simulink model "Zad1"  (R2020b)
settings: Solver=VariableStepAuto  StartTime=0.0  StopTime=0.0  RelTol=1e-3
libraries: CPOiS_SourcesSinks x10, CPOiS_DataManipulation x6, CPOiS_DataManipulation_DataTypeConversion x4, CPOiS_LinearTransforms x2, CPOiS_Filters x2, CPOiS_DataManipulation_IntroduceNoise x1, CPOiS_General x1
settings Model: Creator=Krystian  LastModifiedBy=Krystian

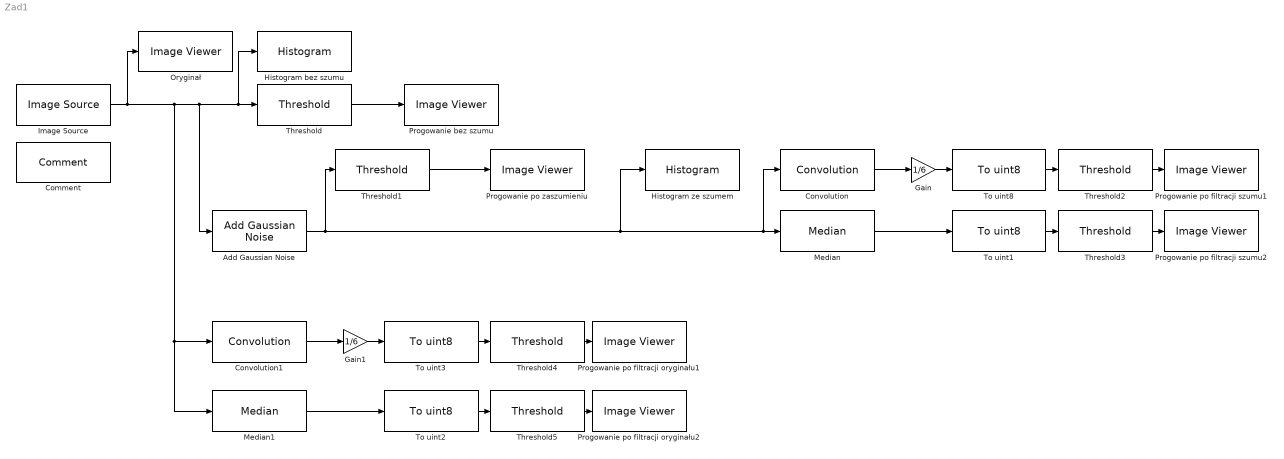
== system Zad1 ==
  Add Gaussian Noise : CPOiS_DataManipulation_IntroduceNoise/Add Gaussian Noise  Mean=0  Variance=1
      settings: SourceProductName=CPOiS - Digital image and signal processing
  Comment : CPOiS_General/Comment
      settings: SourceProductName=CPOiS - Digital image and signal processing
  Convolution : CPOiS_LinearTransforms/Convolution  ConvolutionMatrix=[0,1,0;1,2,1;0,1,0]
      settings: SourceProductName=CPOiS - Digital image and signal processing
  Convolution1 : CPOiS_LinearTransforms/Convolution  ConvolutionMatrix=[0,1,0;1,2,1;0,1,0]
      settings: SourceProductName=CPOiS - Digital image and signal processing
  Gain : Gain  Gain=1/6
  Gain1 : Gain  Gain=1/6
  Histogram bez szumu : CPOiS_SourcesSinks/Histogram
      settings: SourceProductName=CPOiS - Digital image and signal processing
  Histogram ze szumem : CPOiS_SourcesSinks/Histogram
      settings: SourceProductName=CPOiS - Digital image and signal processing
  Image Source : CPOiS_SourcesSinks/Image Source  FileSelection=cameraman.tif
      settings: SourceProductName=CPOiS - Digital image and signal processing
  Median : CPOiS_Filters/Median  MaskSize=3 x 3
      settings: SourceProductName=CPOiS - Digital image and signal processing
  Median1 : CPOiS_Filters/Median  MaskSize=3 x 3
      settings: SourceProductName=CPOiS - Digital image and signal processing
  Oryginał : CPOiS_SourcesSinks/Image Viewer
      settings: SourceProductName=CPOiS - Digital image and signal processing
  Progowanie bez szumu : CPOiS_SourcesSinks/Image Viewer
      settings: SourceProductName=CPOiS - Digital image and signal processing
  Progowanie po filtracji oryginału1 : CPOiS_SourcesSinks/Image Viewer
      settings: SourceProductName=CPOiS - Digital image and signal processing
  Progowanie po filtracji oryginału2 : CPOiS_SourcesSinks/Image Viewer
      settings: SourceProductName=CPOiS - Digital image and signal processing
  Progowanie po filtracji szumu1 : CPOiS_SourcesSinks/Image Viewer
      settings: SourceProductName=CPOiS - Digital image and signal processing
  Progowanie po filtracji szumu2 : CPOiS_SourcesSinks/Image Viewer
      settings: SourceProductName=CPOiS - Digital image and signal processing
  "Progowanie po zaszumieniu " : CPOiS_SourcesSinks/Image Viewer
      settings: SourceProductName=CPOiS - Digital image and signal processing
  Threshold{,1..5} (6 alike) : CPOiS_DataManipulation/Threshold  Threshold=30
      settings: SourceProductName=CPOiS - Digital image and signal processing
  To uint{1..3,8} (4 alike) : CPOiS_DataManipulation_DataTypeConversion/To uint8
      settings: SourceProductName=CPOiS - Digital image and signal processing
  wires:
  Threshold2/1 -> Progowanie po filtracji szumu1/1
  Threshold4/1 -> Progowanie po filtracji oryginału1/1
  Threshold5/1 -> Progowanie po filtracji oryginału2/1
  Image Source/1 -> Oryginał/1, Median1/1, Convolution1/1, Histogram bez szumu/1, Threshold/1, Add Gaussian Noise/1
  Threshold1/1 -> "Progowanie po zaszumieniu "/1
  Gain1/1 -> To uint3/1
  Median1/1 -> To uint2/1
  To uint2/1 -> Threshold5/1
  Convolution1/1 -> Gain1/1
  To uint3/1 -> Threshold4/1
  To uint8/1 -> Threshold2/1
  To uint1/1 -> Threshold3/1
  Threshold3/1 -> Progowanie po filtracji szumu2/1
  Convolution/1 -> Gain/1
  Median/1 -> To uint1/1
  Gain/1 -> To uint8/1
  Add Gaussian Noise/1 -> Convolution/1, Median/1, Histogram ze szumem/1, Threshold1/1
  Threshold/1 -> Progowanie bez szumu/1
